simulink model "EsquemasModulacion_VersionR2016b"  (R2018b)
settings: Solver=ode5  StartTime=0.0  StopTime=30-Tsampling  FixedStep=Tsampling  RelTol=1e-3
values from neighbouring files (symbols this model uses):
  AmplitudPort = AmplitudSignal/indicMod    (= 2)    [ConfigParametros_simulacion.m]
  AmplitudSignal = 1    [ConfigParametros_simulacion.m]
  Es = Eb    (= 2)    [ConfigParametros_simulacion.m]
  Fp = FrecMax*4    (= 4000)    [ConfigParametros_simulacion.m]
  Fp1 = 2*Rs    (= 2000)    [ConfigParametros_simulacion.m]
  Fp2 = 3*Rs    (= 3000)    [ConfigParametros_simulacion.m]
  Rb = FrecMax    (= 1000)    [ConfigParametros_simulacion.m]
  Ts = Tb    (= 0.001)    [ConfigParametros_simulacion.m]
  Tsampling = Tp/100    (= 2.5e-06)    [ConfigParametros_simulacion.m]
libraries: dspsrcs4 x6, commrandsrc3 x1, commdigbbndpm3 x1
settings Model: Creator=lukit  LastModifiedBy=lukit
settings CodeAppCC: StateflowObjectComments=on

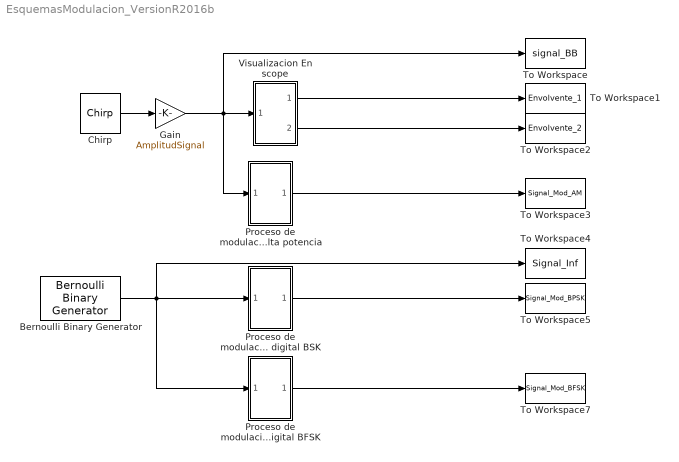
== system EsquemasModulacion_VersionR2016b ==
  Bernoulli Binary Generator : commrandsrc3/Bernoulli Binary Generator  ProbabilityOfZero=0.5  SeedSource=Auto  Seed=0  SampleTime=1/Rb  SamplesPerFrame=1  OutputDataType=double  SimulateUsing=Interpreted execution
      settings: SourceProductName=Communications Toolbox
  Chirp : dspsrcs4/Chirp  sweep=Linear  mode=Unidirectional  f0=Finic  f1=FrecMax  t1=tiemp  Tsweep=tiemp  phase=pi/2  Ts=Tsampling  spf=1  datatype=Double  OutputFrames=off
      settings: SourceProductName=DSP System Toolbox
  Gain : Gain  Gain=AmplitudSignal
  Proceso de modulacion AM con Portadora de alta potencia : Subsystem
  Proceso de modulacion digital BFSK : Subsystem
  Proceso de modulacion digital BSK : Subsystem
  To Workspace : ToWorkspace  VariableName=signal_BB  SampleTime=Tsampling
      settings: Save2DSignal=2-D array (concatenate along first dimension)
  To Workspace1 : ToWorkspace  VariableName=Envolvente_1  SampleTime=Tsampling
      settings: Save2DSignal=2-D array (concatenate along first dimension)
  To Workspace2 : ToWorkspace  VariableName=Envolvente_2  SampleTime=Tsampling
      settings: Save2DSignal=2-D array (concatenate along first dimension)
  To Workspace3 : ToWorkspace  VariableName=Signal_Mod_AM  SampleTime=Tsampling
      settings: Save2DSignal=2-D array (concatenate along first dimension)
  To Workspace4 : ToWorkspace  VariableName=Signal_Inf  SampleTime=Tsampling
      settings: Save2DSignal=2-D array (concatenate along first dimension)
  To Workspace5 : ToWorkspace  VariableName=Signal_Mod_BPSK  SampleTime=Tsampling
      settings: Save2DSignal=2-D array (concatenate along first dimension)
  To Workspace7 : ToWorkspace  VariableName=Signal_Mod_BFSK  SampleTime=Tsampling
      settings: Save2DSignal=2-D array (concatenate along first dimension)
  Visualizacion En scope : Subsystem
  wires:
  Visualizacion En scope/1(Out1) -> To Workspace1/1
  Visualizacion En scope/2(Out2) -> To Workspace2/1
  Proceso de modulacion AM con Portadora de alta potencia/1(Out1) -> To Workspace3/1
  Chirp/1 -> Gain/1
  Gain/1 -> To Workspace/1, Visualizacion En scope/1(In1), Proceso de modulacion AM con Portadora de alta potencia/1(In1)
  Bernoulli Binary Generator/1 -> Proceso de modulacion digital BSK/1(In1), To Workspace4/1, Proceso de modulacion digital BFSK/1(In1)
  Proceso de modulacion digital BSK/1(Out1) -> To Workspace5/1
  Proceso de modulacion digital BFSK/1(Out1) -> To Workspace7/1

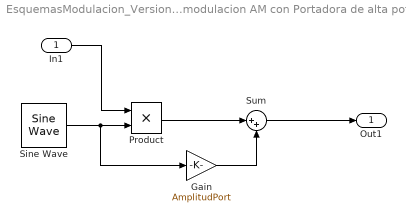
== system EsquemasModulacion_VersionR2016b/Proceso de modulacion AM con Portadora de alta potencia ==
  In1 : Inport
  Gain : Gain  Gain=AmplitudPort
  Product : Product
  Sine Wave : dspsrcs4/Sine Wave  Amplitude=1  Frequency=Fp  Phase=pi/2  SampleMode=Discrete  OutComplex=Real  CompMethod=Trigonometric fcn  TableSize=Speed  SampleTime=Tsampling  SamplesPerFrame=1  ResetState=Restart at time zero  OutputFrames=off  dataType=double  wordLen=16  udDataType=sfix(16)  fracBitsMode=Best precision  numFracBits=15  OutDataTypeStr=double  LastOutDataTypeStr=double
  Sum : Sum  Inputs=|++
  Out1 : Outport
  wires:
  Product/1 -> Sum/1
  Sine Wave/1 -> Gain/1, Product/2
  Sum/1 -> Out1/1
  In1/1 -> Product/1
  Gain/1 -> Sum/2

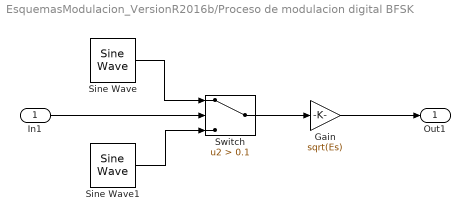
== system EsquemasModulacion_VersionR2016b/Proceso de modulacion digital BFSK ==
  In1 : Inport
  Gain : Gain  Gain=sqrt(Es)
  Sine Wave : dspsrcs4/Sine Wave  Amplitude=sqrt(2/Ts)  Frequency=Fp1  Phase=pi/2  SampleMode=Discrete  OutComplex=Real  CompMethod=Trigonometric fcn  TableSize=Speed  SampleTime=Tsampling  SamplesPerFrame=1  ResetState=Restart at time zero  OutputFrames=off  dataType=double  wordLen=16  udDataType=sfix(16)  fracBitsMode=Best precision  numFracBits=15  OutDataTypeStr=double  LastOutDataTypeStr=double
  Sine Wave1 : dspsrcs4/Sine Wave  Amplitude=sqrt(2/Ts)  Frequency=Fp2  Phase=pi/2  SampleMode=Discrete  OutComplex=Real  CompMethod=Trigonometric fcn  TableSize=Speed  SampleTime=Tsampling  SamplesPerFrame=1  ResetState=Restart at time zero  OutputFrames=off  dataType=double  wordLen=16  udDataType=sfix(16)  fracBitsMode=Best precision  numFracBits=15  OutDataTypeStr=double  LastOutDataTypeStr=double
  Switch : Switch  Criteria=u2 > Threshold  Threshold=0.1
  Out1 : Outport
  wires:
  Sine Wave/1 -> Switch/1
  Sine Wave1/1 -> Switch/3
  Switch/1 -> Gain/1
  In1/1 -> Switch/2
  Gain/1 -> Out1/1

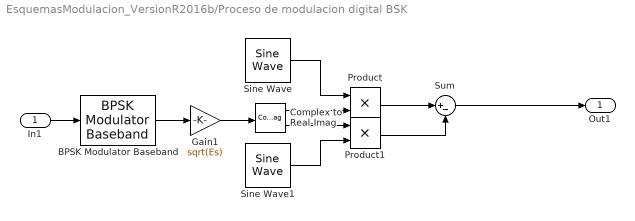
== system EsquemasModulacion_VersionR2016b/Proceso de modulacion digital BSK ==
  In1 : Inport
  BPSK Modulator Baseband : commdigbbndpm3/BPSK Modulator Baseband  Ph=0  outDtype=double  outWordLen=16  outUDDataType=sfix(16)  outFracLenMode=Best precision  outFracLen=15  outDataTypeStr=double  outLastDataTypeStr=double
      settings: SourceProductName=Communications Toolbox
  Complex to Real-Imag : ComplexToRealImag
  Gain1 : Gain  Gain=sqrt(Es)
  Product : Product
  Product1 : Product
  Sine Wave : dspsrcs4/Sine Wave  Amplitude=sqrt(2/Ts)  Frequency=Fp  Phase=pi/2  SampleMode=Discrete  OutComplex=Real  CompMethod=Trigonometric fcn  TableSize=Speed  SampleTime=Tsampling  SamplesPerFrame=1  ResetState=Restart at time zero  OutputFrames=off  dataType=double  wordLen=16  udDataType=sfix(16)  fracBitsMode=Best precision  numFracBits=15  OutDataTypeStr=double  LastOutDataTypeStr=double
  Sine Wave1 : dspsrcs4/Sine Wave  Amplitude=sqrt(2/Ts)  Frequency=Fp  Phase=pi/2  SampleMode=Discrete  OutComplex=Real  CompMethod=Trigonometric fcn  TableSize=Speed  SampleTime=Tsampling  SamplesPerFrame=1  ResetState=Restart at time zero  OutputFrames=off  dataType=double  wordLen=16  udDataType=sfix(16)  fracBitsMode=Best precision  numFracBits=15  OutDataTypeStr=double  LastOutDataTypeStr=double
  Sum : Sum  Inputs=|+-
  Out1 : Outport
  wires:
  In1/1 -> BPSK Modulator Baseband/1
  Sine Wave1/1 -> Product1/2
  BPSK Modulator Baseband/1 -> Gain1/1
  Product1/1 -> Sum/2
  Sine Wave/1 -> Product/1
  Complex to Real-Imag/1 -> Product/2
  Complex to Real-Imag/2 -> Product1/1
  Gain1/1 -> Complex to Real-Imag/1
  Product/1 -> Sum/1
  Sum/1 -> Out1/1

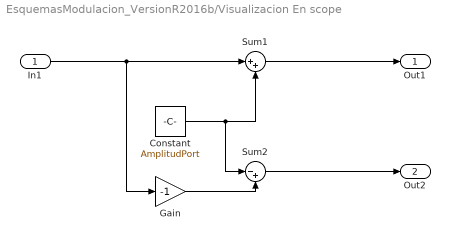
== system EsquemasModulacion_VersionR2016b/Visualizacion En scope ==
  In1 : Inport
  Constant : Constant  Value=AmplitudPort
  Gain : Gain  Gain=-1
  Sum1 : Sum  Inputs=|++
  Sum2 : Sum  Inputs=|-+
  Out1 : Outport
  Out2 : Outport  Port=2
  wires:
  In1/1 -> Sum1/1, Gain/1
  Constant/1 -> Sum2/1, Sum1/2
  Sum1/1 -> Out1/1
  Sum2/1 -> Out2/1
  Gain/1 -> Sum2/2
